simulink model "P5"  (R2020b)
settings: Solver=VariableStepAuto  StartTime=0.0  StopTime=0.004  RelTol=1e-3
settings Model: Creator=stank  LastModifiedBy=stank

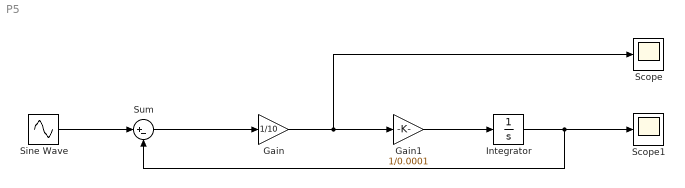
== system P5 ==
  Gain : Gain  Gain=1/10
  Gain1 : Gain  Gain=1/0.0001
  Integrator : Integrator
  Scope : Scope
  Scope1 : Scope
  Sine Wave : Sin  Amplitude=10  Frequency=50  SampleTime=0
  Sum : Sum  Inputs=|+-
  wires:
  Sine Wave/1 -> Sum/1
  Sum/1 -> Gain/1
  Gain/1 -> Scope/1, Gain1/1
  Gain1/1 -> Integrator/1
  Integrator/1 -> Sum/2, Scope1/1
